simulink model "COMPONENT_MDL_Lag_QUAD_and_PEND_with_Ab"  (R2020b)
settings: Solver=ode23t  StartTime=0.0  StopTime=200  FixedStep=0.001  RelTol=1e-5  EnableMultiTasking=on
undefined symbols (not defined in the file or in its folder): P_pend, P_rot, P_veh_no_props
(part 2 of 12)

== matlab function COMPONENT_MDL_Lag_QUAD_and_PEND_with_Ab/bh_6DOF_and_pend/A_and_b ==
  data: I_xx input; A output; I_xy input; I_xz input; I_yy input; I_yz input; I_zz input; Iprop_xx input; Iprop_xy input; Iprop_xz input; Iprop_yy input; Iprop_yz input; Iprop_zz input; Lx_pend input; Ly_pend input; Lz_pend input; Mbz_1 input; Mbz_2 input; Mbz_3 input; Mbz_4 input; THE_X_D input; THE_Y_D input; THE_Z_D input; THE_Phi input; THE_Psi input; THE_Phi_D input; THE_Psi_D input; THE_Theta input; THE_Theta_D input; THE_Phi_pend input; THE_Psi_pend input; THE_Phi_pend_D input; THE_Psi_pend_D input; THE_Theta_pend input; THE_Theta_pend_D input; Tbz_1 input; Tbz_2 input; Tbz_3 input; Tbz_4 input; Tv_Z_pend input; cg_to_mot_H input; cg_to_mot_L input; g input; m input; m_pend input; mprop input; wMOT_1 input; wMOT_2 input; wMOT_3 input; wMOT_4 input; b output
function [A,b] = A_and_b(I_xx,I_xy,I_xz,I_yy,I_yz,I_zz,Iprop_xx,Iprop_xy,Iprop_xz,Iprop_yy,Iprop_yz,Iprop_zz,Lx_pend,Ly_pend,Lz_pend,Mbz_1,Mbz_2,Mbz_3,Mbz_4,THE_X_D,THE_Y_D,THE_Z_D,THE_Phi,THE_Psi,THE_Phi_D,THE_Psi_D,THE_Theta,THE_Theta_D,THE_Phi_pend,THE_Psi_pend,THE_Phi_pend_D,THE_Psi_pend_D,THE_Theta_pend,THE_Theta_pend_D,Tbz_1,Tbz_2,Tbz_3,Tbz_4,Tv_Z_pend,cg_to_mot_H,cg_to_mot_L,g,m,m_pend,mprop,wMOT_1,wMOT_2,wMOT_3,wMOT_4)
%#codegen

%    This function was generated by the Symbolic Math Toolbox version 8.6.
%    11-Jan-2021 14:04:52

